simulink model "test_sim"  (R2023b)
settings: Solver=VariableStepAuto  StartTime=0.0  StopTime=1  RelTol=1e-3
values from neighbouring files (symbols this model uses):
  Ts = 0.01    [grandland.m]    (also in grandland_3.m = 0.02; test.m)
libraries: cstblocks x9
settings Model: Creator=antor  LastModifiedBy=antor

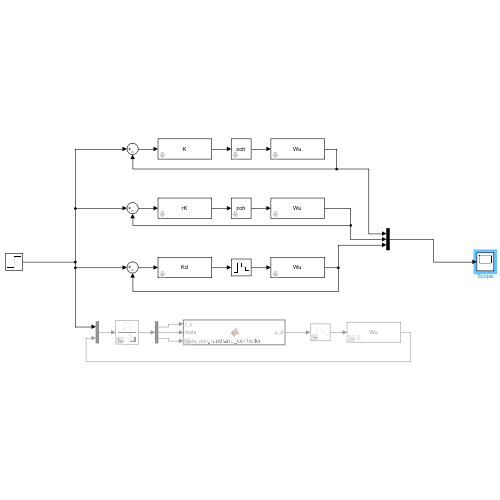
[thumbnail: Simulink's stored preview of the top-level diagram]
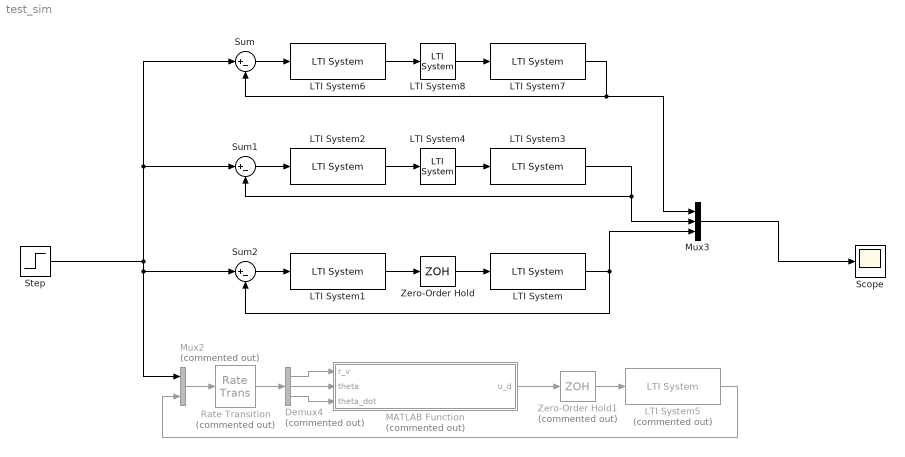
== system test_sim ==
  Demux4 : Demux  Commented=on  Outputs=3
  LTI System : cstblocks/LTI System  sys=Wu  IC=[]  PadeOrder=0
  LTI System1 : cstblocks/LTI System  sys=Kd  IC=[]  PadeOrder=0
  LTI System2 : cstblocks/LTI System  sys=rK  IC=[]  PadeOrder=0
  LTI System3 : cstblocks/LTI System  sys=Wu  IC=[]  PadeOrder=0
  LTI System4 : cstblocks/LTI System  sys=zoh  IC=[]  PadeOrder=0
  LTI System5 : cstblocks/LTI System  Commented=on  sys=Wu  IC=[]  PadeOrder=0
  LTI System6 : cstblocks/LTI System  sys=K  IC=[]  PadeOrder=0
  LTI System7 : cstblocks/LTI System  sys=Wu  IC=[0 0]  PadeOrder=0
  LTI System8 : cstblocks/LTI System  sys=zoh  IC=[]  PadeOrder=0
  MATLAB Function : MATLAB Function  Commented=on  TreatAsAtomicUnit=on
  Mux2 : Mux  Commented=on  Inputs=2
  Mux3 : Mux  Inputs=3
  Rate Transition : RateTransition  Commented=on  OutPortSampleTime=Ts
  Scope : Scope
  Step : Step  Time=0  After=0.1  SampleTime=0
  Sum : Sum  Inputs=|+-
  Sum1 : Sum  Inputs=|+-
  Sum2 : Sum  Inputs=|+-
  Zero-Order Hold : ZeroOrderHold  SampleTime=Ts
  Zero-Order Hold1 : ZeroOrderHold  Commented=on  SampleTime=Ts
  wires:
  LTI System8/1 -> LTI System7/1
  LTI System/1 -> Mux3/3, Sum2/2
  LTI System6/1 -> LTI System8/1
  Zero-Order Hold1/1 -> LTI System5/1
  LTI System3/1 -> Sum1/2, Mux3/2
  Mux3/1 -> Scope/1
  MATLAB Function/1(u_d) -> Zero-Order Hold1/1
  Demux4/1 -> MATLAB Function/1(r_v)
  Rate Transition/1 -> Demux4/1
  Step/1 -> Sum1/1, Sum/1, Sum2/1, Mux2/1
  Demux4/2 -> MATLAB Function/2(theta)
  LTI System7/1 -> Sum/2, Mux3/1
  Demux4/3 -> MATLAB Function/3(theta_dot)
  LTI System5/1 -> Mux2/2
  Mux2/1 -> Rate Transition/1
  Zero-Order Hold/1 -> LTI System/1
  LTI System1/1 -> Zero-Order Hold/1
  LTI System4/1 -> LTI System3/1
  LTI System2/1 -> LTI System4/1
  Sum/1 -> LTI System6/1
  Sum1/1 -> LTI System2/1
  Sum2/1 -> LTI System1/1

== matlab function test_sim/MATLAB Function ==
  settings: updateMethod=DISCRETE
  data: Kd_coeff parameter; r_v input; theta input; theta_dot input; u_d output
function u_d = grandland_controller(Kd_coeff, r_v, theta, theta_dot)

persistent state;
if isempty(state)
    state = zeros(4, 3);
end

state(:, 2:3) = state(:, 1:2);
state(1:3, 1) = [r_v; theta; theta_dot];

u_d = 0;
for i = 1:3
    num = Kd_coeff(i, 1:3);
    u_d = u_d+(num(1)*state(i, 1)+num(2)*state(i, 2)+num(3)*state(i, 3));
end
den = Kd_coeff(i+1, 1:3);
u_d = u_d-den(2)*state(4, 2)-den(3)*state(4, 3);

state(4, 1) = u_d;

end
